simulink model "combined_mdl_wpanel"  (R2024b)
settings: Solver=FixedStepAuto  StartTime=0.0  StopTime=Inf  FixedStep=0.1  MaxStep=1e-3  RelTol=1e-3
model workspace: external: MATLAB File model\combined_mdl_wpanel_wkspc.m (data not in the file)
values from neighbouring files (symbols this model uses):
  sample_period_ms = 100    [combined_mdl_wpanel_wkspc.m]
undefined symbols (not defined in the file or in its folder): DiscIntNeverNeededParam, Serial_Port, Standard_Devices
libraries: simulink x2, sldrtlib x2
settings Model: Creator=apm3  LastModifiedBy=baley
settings HardwareCC: ProdBitPerLong=64  ProdHWDeviceType=Intel->x86-64 (Linux 64)
settings ModelReferenceCC: EnableRefExpFcnMdlSchedulingChecks=on
settings RTWCC: Description=Simulink Desktop Real-Time  SystemTargetFile=sldrt.tlc  TemplateMakefile=sldrt.tmf  RTWCompilerOptimization=on  GPUComputeCapability=3.5
settings CodeAppCC: MaxIdLength=95
settings SimulinkDesktopRealTimeCC: TargetLibSuffix=_sldrt.a  TargetPreCompLibLocation=/home/baley/matlab/R2024b/toolbox/sldrt/lib/glnxa64  ParMdlRefBuildCompliant=on

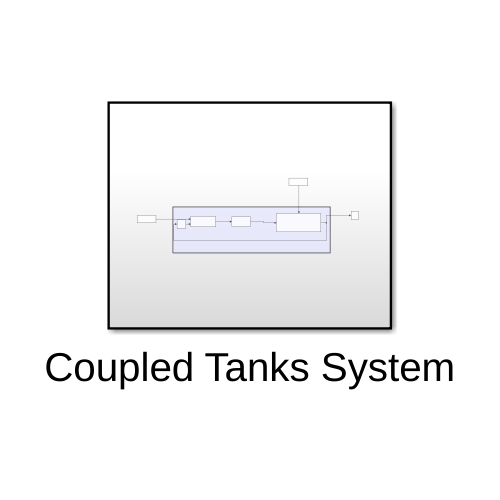
[thumbnail: Simulink's stored preview of the top-level diagram]
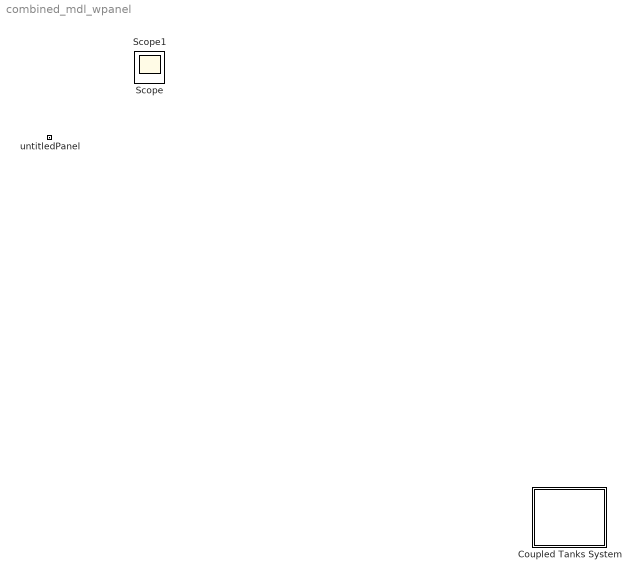
== system combined_mdl_wpanel ==
  Coupled Tanks System : Subsystem
  untitledPanel : Subsystem  Tag=HiddenForWebPanel  IsWebBlockPanel=on
  Scope : Scope
  Scope1 : Scope

== system combined_mdl_wpanel/Coupled Tanks System ==
  note: System
  Controller : Subsystem
  Disturbance : Subsystem
      settings: PortSchema="{\"entries\":[{\"content\":{\"sides\":[{\"content\":{},\"type\":\"ConnectorPlacement.EquallySpacedRectSide\",\"uuid\":\"af3cbaf0-e8cb-4094-98c2-a613e4267cda\"},{\"content\":{\"side\":\"RIGHT\"},\"type\":\"ConnectorPlacement.EquallySpacedRectSide\",\"uuid\":\"ca2a579d-f09d-4edc-8bb1-bcf470cd6e52\"},{\"content\":{\"side\":\"TOP\"},\"type\":\"ConnectorPlacement.EquallySpacedRectSide\",\"uuid\":\"8ccf8dff-0f76-45f4-a120-4302248ce1f5\"},{\"content\":{\"connectorIds\":[\"Out1\"],\"side\":\"BOTTOM\"},\"type\":\"ConnectorPlacement.EquallySpacedRectSide\",\"uuid\":\"e11fb4df-eb62-4915-8053-08a1cec1e132\"}]},\"type\":\"ConnectorPlacement.EquallySpacedConnector\",\"uuid\":\"71d40907-b541-4068-8366-dc0e6cb107c2\"}],\"packageUris\":[\"http://schema.mathworks.com/mf0/Connector/R2020b\"],\"version\":\"1.0\"}"
  Feedback : Subsystem
  Output Scope : Scope
  Plant - Coupled Tanks : Subsystem
      settings: PortSchema="{\"entries\":[{\"content\":{\"sides\":[{\"content\":{\"connectorIds\":[\"In1\"]},\"type\":\"ConnectorPlacement.EquallySpacedRectSide\",\"uuid\":\"4813ac87-9876-4add-8b68-135f8eb15e0b\"},{\"content\":{\"connectorIds\":[\"Out1\"],\"side\":\"RIGHT\"},\"type\":\"ConnectorPlacement.EquallySpacedRectSide\",\"uuid\":\"8da6c8ab-654d-4da4-994c-054b6b84e45c\"},{\"content\":{\"connectorIds\":[\"In2\"],\"side\":\"TOP\"},\"type\":\"ConnectorPlacement.EquallySpacedRectSide\",\"uuid\":\"bc816fc0-ca42-463e-8b06-f8322ae18973\"},{\"content\":{\"side\":\"BOTTOM\"},\"type\":\"ConnectorPlacement.EquallySpacedRectSide\",\"uuid\":\"34484812-162f-4898-b397-ade1a8525c9d\"}]},\"type\":\"ConnectorPlacement.EquallySpacedConnector\",\"uuid\":\"89f4005a-211d-406b-8623-1dc8ebdf98c9\"}],\"packageUris\":[\"http://schema.mathworks.com/mf0/Connector/R2020b\"],\"version\":\"1.0\"}"
  Reference Signal : Subsystem
  Unit Delay : UnitDelay  SampleTime=-1  HasFrameUpgradeWarning=on
  wires:
  Controller/1(Controller Output) -> Plant - Coupled Tanks/1(In2)
  Plant - Coupled Tanks/1(Output Variable) -> Output Scope/1, Unit Delay/1  "measured"
  Disturbance/1(Disturbance Signal) -> Plant - Coupled Tanks/2(Disturbance)
  Reference Signal/1(Reference Signal) -> Feedback/1(Signal)
  Feedback/1(Output) -> Controller/1(Input)
  Unit Delay/1 -> Feedback/2(Output Variable)

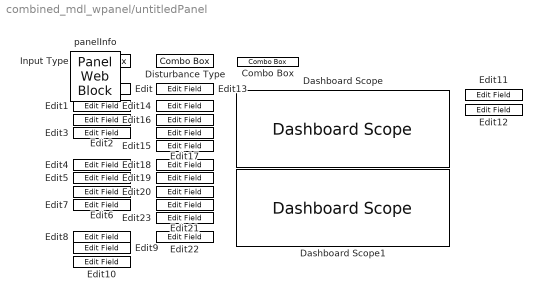
== system combined_mdl_wpanel/untitledPanel ==
  Combo Box : ComboBox  Tag=HiddenForWebPanel  PanelInfo="{\"height\":19,\"left\":400,\"panelId\":\"panelId-cfd753c6-38f0-4228-886e-ef133e3498b9\",\"top\":46,\"type\":\"panelChild\",\"version\":\"2019b\",\"width\":134,\"zIndex\":1500004}"  LabelPosition=Hide  SelectedLabel=Actual Plant
      settings: Values={{'Simulated Plant', 'Actual Plant'}, [0 1]}
  Dashboard Scope : DashboardScope  Tag=HiddenForWebPanel  PanelInfo="{\"height\":168,\"left\":397,\"panelId\":\"panelId-cfd753c6-38f0-4228-886e-ef133e3498b9\",\"top\":119,\"type\":\"panelChild\",\"version\":\"2019b\",\"width\":467,\"zIndex\":1500010}"
  Dashboard Scope1 : DashboardScope  Tag=HiddenForWebPanel  PanelInfo="{\"height\":168,\"left\":397,\"panelId\":\"panelId-cfd753c6-38f0-4228-886e-ef133e3498b9\",\"top\":292,\"type\":\"panelChild\",\"version\":\"2019b\",\"width\":467,\"zIndex\":1500058}"
  Disturbance Type : ComboBox  Tag=HiddenForWebPanel  PanelInfo="{\"height\":29,\"left\":222,\"panelId\":\"panelId-cfd753c6-38f0-4228-886e-ef133e3498b9\",\"top\":40,\"type\":\"panelChild\",\"version\":\"2019b\",\"width\":125,\"zIndex\":1500006}"  LabelPosition=Hide  SelectedLabel=None
      settings: Values={{'None', 'Constant', 'Sine', 'Square', 'Chirp', 'Arbitrary'}, [1 2 3 4 5 6]}
  Edit : EditField  Tag=HiddenForWebPanel  PanelInfo="{\"height\":24,\"left\":40,\"panelId\":\"panelId-cfd753c6-38f0-4228-886e-ef133e3498b9\",\"top\":103,\"type\":\"panelChild\",\"version\":\"2019b\",\"width\":125,\"zIndex\":1500018}"  ShowInitialText=on  Alignment=Left
  Edit1 : EditField  Tag=HiddenForWebPanel  PanelInfo="{\"height\":24,\"left\":40,\"panelId\":\"panelId-cfd753c6-38f0-4228-886e-ef133e3498b9\",\"top\":141,\"type\":\"panelChild\",\"version\":\"2019b\",\"width\":125,\"zIndex\":1500008}"  ShowInitialText=on  Alignment=Left
  Edit10 : EditField  Tag=HiddenForWebPanel  PanelInfo="{\"height\":24,\"left\":40,\"panelId\":\"panelId-cfd753c6-38f0-4228-886e-ef133e3498b9\",\"top\":482,\"type\":\"panelChild\",\"version\":\"2019b\",\"width\":125,\"zIndex\":1500040}"  ShowInitialText=on  Alignment=Left
  Edit11 : EditField  Tag=HiddenForWebPanel  PanelInfo="{\"height\":24,\"left\":900,\"panelId\":\"panelId-cfd753c6-38f0-4228-886e-ef133e3498b9\",\"top\":116,\"type\":\"panelChild\",\"version\":\"2019b\",\"width\":125,\"zIndex\":1500046}"  ShowInitialText=on  Alignment=Left
  Edit12 : EditField  Tag=HiddenForWebPanel  PanelInfo="{\"height\":24,\"left\":900,\"panelId\":\"panelId-cfd753c6-38f0-4228-886e-ef133e3498b9\",\"top\":149,\"type\":\"panelChild\",\"version\":\"2019b\",\"width\":125,\"zIndex\":1500048}"  ShowInitialText=on  Alignment=Left
  Edit13 : EditField  Tag=HiddenForWebPanel  PanelInfo="{\"height\":24,\"left\":222,\"panelId\":\"panelId-cfd753c6-38f0-4228-886e-ef133e3498b9\",\"top\":103,\"type\":\"panelChild\",\"version\":\"2019b\",\"width\":125,\"zIndex\":1500024}"  ShowInitialText=on  Alignment=Left
  Edit14 : EditField  Tag=HiddenForWebPanel  PanelInfo="{\"height\":24,\"left\":222,\"panelId\":\"panelId-cfd753c6-38f0-4228-886e-ef133e3498b9\",\"top\":141,\"type\":\"panelChild\",\"version\":\"2019b\",\"width\":125,\"zIndex\":1500042}"  ShowInitialText=on  Alignment=Left
  Edit15 : EditField  Tag=HiddenForWebPanel  PanelInfo="{\"height\":24,\"left\":222,\"panelId\":\"panelId-cfd753c6-38f0-4228-886e-ef133e3498b9\",\"top\":228,\"type\":\"panelChild\",\"version\":\"2019b\",\"width\":125,\"zIndex\":1500028}"  ShowInitialText=on  Alignment=Left
  Edit16 : EditField  Tag=HiddenForWebPanel  PanelInfo="{\"height\":24,\"left\":222,\"panelId\":\"panelId-cfd753c6-38f0-4228-886e-ef133e3498b9\",\"top\":171,\"type\":\"panelChild\",\"version\":\"2019b\",\"width\":125,\"zIndex\":1500020}"  ShowInitialText=on  Alignment=Left
  Edit17 : EditField  Tag=HiddenForWebPanel  PanelInfo="{\"height\":24,\"left\":222,\"panelId\":\"panelId-cfd753c6-38f0-4228-886e-ef133e3498b9\",\"top\":200,\"type\":\"panelChild\",\"version\":\"2019b\",\"width\":125,\"zIndex\":1500002}"  ShowInitialText=on  Alignment=Left
  Edit18 : EditField  Tag=HiddenForWebPanel  PanelInfo="{\"height\":24,\"left\":222,\"panelId\":\"panelId-cfd753c6-38f0-4228-886e-ef133e3498b9\",\"top\":269,\"type\":\"panelChild\",\"version\":\"2019b\",\"width\":125,\"zIndex\":1500030}"  ShowInitialText=on  Alignment=Left
  Edit19 : EditField  Tag=HiddenForWebPanel  PanelInfo="{\"height\":24,\"left\":222,\"panelId\":\"panelId-cfd753c6-38f0-4228-886e-ef133e3498b9\",\"top\":298,\"type\":\"panelChild\",\"version\":\"2019b\",\"width\":125,\"zIndex\":1500032}"  ShowInitialText=on  Alignment=Left
  Edit2 : EditField  Tag=HiddenForWebPanel  PanelInfo="{\"height\":24,\"left\":40,\"panelId\":\"panelId-cfd753c6-38f0-4228-886e-ef133e3498b9\",\"top\":171,\"type\":\"panelChild\",\"version\":\"2019b\",\"width\":125,\"zIndex\":1500026}"  ShowInitialText=on  Alignment=Left
  Edit20 : EditField  Tag=HiddenForWebPanel  PanelInfo="{\"height\":24,\"left\":222,\"panelId\":\"panelId-cfd753c6-38f0-4228-886e-ef133e3498b9\",\"top\":328,\"type\":\"panelChild\",\"version\":\"2019b\",\"width\":125,\"zIndex\":1500044}"  ShowInitialText=on  Alignment=Left
  Edit21 : EditField  Tag=HiddenForWebPanel  PanelInfo="{\"height\":24,\"left\":222,\"panelId\":\"panelId-cfd753c6-38f0-4228-886e-ef133e3498b9\",\"top\":357,\"type\":\"panelChild\",\"version\":\"2019b\",\"width\":125,\"zIndex\":1500012}"  ShowInitialText=on  Alignment=Left
  Edit22 : EditField  Tag=HiddenForWebPanel  PanelInfo="{\"height\":24,\"left\":222,\"panelId\":\"panelId-cfd753c6-38f0-4228-886e-ef133e3498b9\",\"top\":428,\"type\":\"panelChild\",\"version\":\"2019b\",\"width\":125,\"zIndex\":1500014}"  ShowInitialText=on  Alignment=Left
  Edit23 : EditField  Tag=HiddenForWebPanel  PanelInfo="{\"height\":24,\"left\":222,\"panelId\":\"panelId-cfd753c6-38f0-4228-886e-ef133e3498b9\",\"top\":385,\"type\":\"panelChild\",\"version\":\"2019b\",\"width\":125,\"zIndex\":1500034}"  ShowInitialText=on  Alignment=Left
  Edit3 : EditField  Tag=HiddenForWebPanel  PanelInfo="{\"height\":24,\"left\":40,\"panelId\":\"panelId-cfd753c6-38f0-4228-886e-ef133e3498b9\",\"top\":200,\"type\":\"panelChild\",\"version\":\"2019b\",\"width\":125,\"zIndex\":1500016}"  ShowInitialText=on  Alignment=Left
  Edit4 : EditField  Tag=HiddenForWebPanel  PanelInfo="{\"height\":24,\"left\":40,\"panelId\":\"panelId-cfd753c6-38f0-4228-886e-ef133e3498b9\",\"top\":269,\"type\":\"panelChild\",\"version\":\"2019b\",\"width\":125,\"zIndex\":1500036}"  ShowInitialText=on  Alignment=Left
  Edit5 : EditField  Tag=HiddenForWebPanel  PanelInfo="{\"height\":24,\"left\":40,\"panelId\":\"panelId-cfd753c6-38f0-4228-886e-ef133e3498b9\",\"top\":298,\"type\":\"panelChild\",\"version\":\"2019b\",\"width\":125,\"zIndex\":1500022}"  ShowInitialText=on  Alignment=Left
  Edit6 : EditField  Tag=HiddenForWebPanel  PanelInfo="{\"height\":24,\"left\":40,\"panelId\":\"panelId-cfd753c6-38f0-4228-886e-ef133e3498b9\",\"top\":328,\"type\":\"panelChild\",\"version\":\"2019b\",\"width\":125,\"zIndex\":1500038}"  ShowInitialText=on  Alignment=Left
  Edit7 : EditField  Tag=HiddenForWebPanel  PanelInfo="{\"height\":24,\"left\":40,\"panelId\":\"panelId-cfd753c6-38f0-4228-886e-ef133e3498b9\",\"top\":357,\"type\":\"panelChild\",\"version\":\"2019b\",\"width\":125,\"zIndex\":1500050}"  ShowInitialText=on  Alignment=Left
  Edit8 : EditField  Tag=HiddenForWebPanel  PanelInfo="{\"height\":24,\"left\":40,\"panelId\":\"panelId-cfd753c6-38f0-4228-886e-ef133e3498b9\",\"top\":428,\"type\":\"panelChild\",\"version\":\"2019b\",\"width\":125,\"zIndex\":1500054}"  ShowInitialText=on  Alignment=Left
  Edit9 : EditField  Tag=HiddenForWebPanel  PanelInfo="{\"height\":24,\"left\":40,\"panelId\":\"panelId-cfd753c6-38f0-4228-886e-ef133e3498b9\",\"top\":452,\"type\":\"panelChild\",\"version\":\"2019b\",\"width\":125,\"zIndex\":1500056}"  ShowInitialText=on  Alignment=Left
  Input Type : ComboBox  Tag=HiddenForWebPanel  PanelInfo="{\"height\":29,\"left\":40,\"panelId\":\"panelId-cfd753c6-38f0-4228-886e-ef133e3498b9\",\"top\":40,\"type\":\"panelChild\",\"version\":\"2019b\",\"width\":125,\"zIndex\":1500052}"  LabelPosition=Hide  SelectedLabel=None
      settings: Values={{'None', 'Constant', 'Sine', 'Square', 'Chirp', 'Arbitrary'}, [1 2 3 4 5 6]}
  panelInfo : PanelWebBlock  Tag=HiddenForWebPanel  PanelInfo="{\"compacted\":false,\"height\":557,\"isActiveTab\":true,\"left\":13,\"name\":\"Panel\",\"panelId\":\"panelId-cfd753c6-38f0-4228-886e-ef133e3498b9\",\"popoutData\":{\"height\":1161,\"left\":-1,\"maximized\":false,\"top\":-8,\"width\":1922},\"popoutMode\":\"windowHidden\",\"tabIndex\":0,\"tabbedSetId\":\"tabbedSet6961756998\",\"top\":50,\"type\":\"panel\",\"version\":\"2019b\",\"visible\":true,\"width\":1077,\"zIndex\":1500002}"  PanelSnapshot=<binary blob, 93600 chars, not shown>

== system combined_mdl_wpanel/Coupled Tanks System/Controller ==
  Input : Inport
  To Workspace : ToWorkspace  VariableName=control_output  SaveFormat=Timeseries  SampleTime=-1
  Controller Output : Outport
  wires:
  Input/1 -> To Workspace/1, Controller Output/1

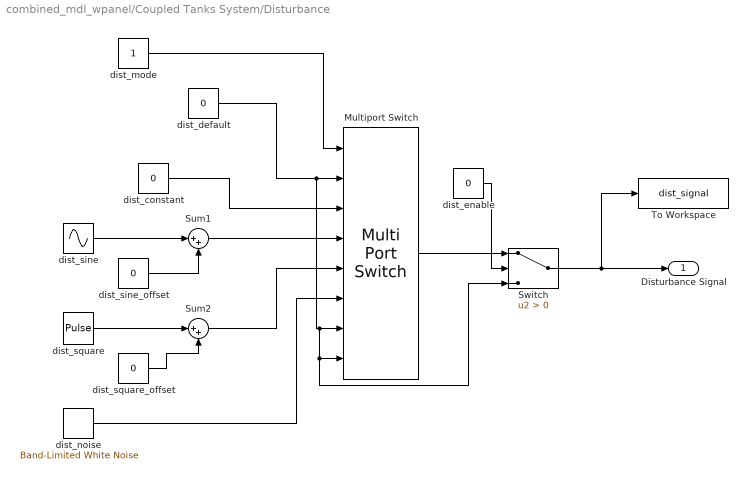
== system combined_mdl_wpanel/Coupled Tanks System/Disturbance ==
  Multiport Switch : MultiPortSwitch  Inputs=6  DataPortForDefault=Additional data port  SaturateOnIntegerOverflow=off  InputSameDT=off
  Sum1 : Sum  Inputs=|++
  Sum2 : Sum  Inputs=|++
  Switch : Switch  Criteria=u2 > Threshold  SaturateOnIntegerOverflow=off  InputSameDT=off
  To Workspace : ToWorkspace  VariableName=dist_signal  SaveFormat=Timeseries  SampleTime=-1
  dist_constant : Constant  Value=0
  dist_default : Constant  Value=0
  dist_enable : Constant  Value=0
  dist_mode : Constant
  dist_noise : simulink/Sources/Band-Limited White Noise  Cov=0  Ts=0.1  seed=[23341]
  dist_sine : Sin  Amplitude=0  Frequency=0  SampleTime=0
  dist_sine_offset : Constant  Value=0
  dist_square : DiscretePulseGenerator  PulseType=Time based  Amplitude=0  Period=1  PulseWidth=50
  dist_square_offset : Constant  Value=0
  Disturbance Signal : Outport
  wires:
  dist_sine/1 -> Sum1/1
  dist_sine_offset/1 -> Sum1/2
  dist_square_offset/1 -> Sum2/2
  dist_square/1 -> Sum2/1
  dist_mode/1 -> Multiport Switch/1
  dist_constant/1 -> Multiport Switch/3
  Sum1/1 -> Multiport Switch/4
  Sum2/1 -> Multiport Switch/5
  dist_noise/1 -> Multiport Switch/6
  Switch/1 -> To Workspace/1, Disturbance Signal/1
  dist_default/1 -> Multiport Switch/8, Switch/3, Multiport Switch/7, Multiport Switch/2
  Multiport Switch/1 -> Switch/1
  dist_enable/1 -> Switch/2

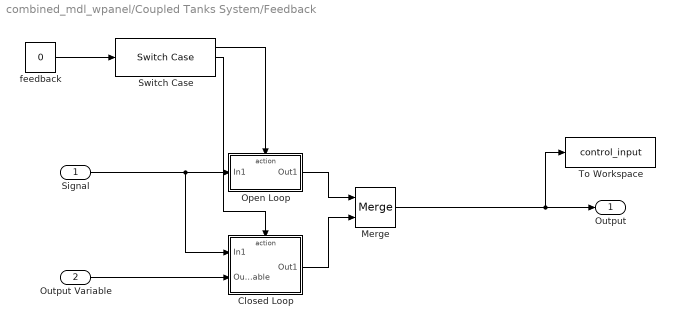
== system combined_mdl_wpanel/Coupled Tanks System/Feedback ==
  Signal : Inport
  Output Variable : Inport  Port=2
  Closed Loop : Subsystem  TreatAsAtomicUnit=on
  Merge : Merge
  Open Loop : Subsystem  TreatAsAtomicUnit=on
  Switch Case : SwitchCase  CaseConditions={0,1}
  To Workspace : ToWorkspace  VariableName=control_input  SaveFormat=Timeseries  SampleTime=-1
  feedback : Constant  Value=0
  Output : Outport
  wires:
  Output Variable/1 -> Closed Loop/2(Output Variable)
  Switch Case/1 -> Open Loop/Action
  Merge/1 -> To Workspace/1, Output/1
  Closed Loop/1(Out1) -> Merge/2
  feedback/1 -> Switch Case/1
  Open Loop/1(Out1) -> Merge/1
  Signal/1 -> Closed Loop/1(In1), Open Loop/1(In1)
  Switch Case/2 -> Closed Loop/Action

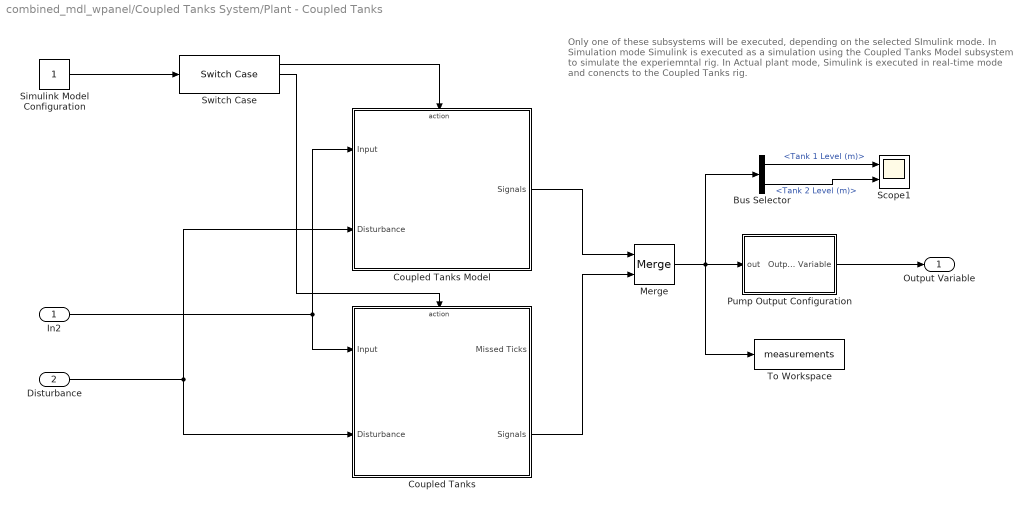
== system combined_mdl_wpanel/Coupled Tanks System/Plant - Coupled Tanks ==
  note: Only one of these subsystems will be executed, depending on the selected SImulink mode.
      |
      | In Simulation mode Simulink is executed as a simulation using the Coupled Tanks Model subsystem to simulate the experiemntal rig.
      |
      | In Actual plant mode, Simulink is executed in real-time mode and conencts to the Coupled Tanks rig.
  In2 : Inport
  Disturbance : Inport  Port=2
  Bus Selector : BusSelector  OutputSignals=Tank 1 Level (m),Tank 2 Level (m)
  Coupled Tanks : Subsystem  TreatAsAtomicUnit=on
  Coupled Tanks Model : Subsystem  TreatAsAtomicUnit=on
  Merge : Merge
  Pump Output Configuration : Subsystem
  Scope1 : Scope  NumInputPorts=2
  Simulink Model Configuration : Constant  OutMin=0  OutMax=1  OutDataTypeStr=int8
  Switch Case : SwitchCase  CaseConditions={0, 1}
  To Workspace : ToWorkspace  VariableName=measurements  SaveFormat=Timeseries  SampleTime=-1
  Output Variable : Outport
  wires:
  Switch Case/2 -> Coupled Tanks/Action
  Switch Case/1 -> Coupled Tanks Model/Action
  In2/1 -> Coupled Tanks/1(Input), Coupled Tanks Model/1(Input)
  Simulink Model Configuration/1 -> Switch Case/1
  Coupled Tanks Model/1(Signals) -> Merge/1
  Coupled Tanks/2(Signals) -> Merge/2
  Merge/1 -> To Workspace/1, Bus Selector/1, Pump Output Configuration/1(out)
  Disturbance/1 -> Coupled Tanks Model/2(Disturbance), Coupled Tanks/2(Disturbance)
  Pump Output Configuration/1(Output Variable) -> Output Variable/1
  Bus Selector/1 -> Scope1/1  "<Tank 1 Level (m)>"
  Bus Selector/2 -> Scope1/2  "<Tank 2 Level (m)>"

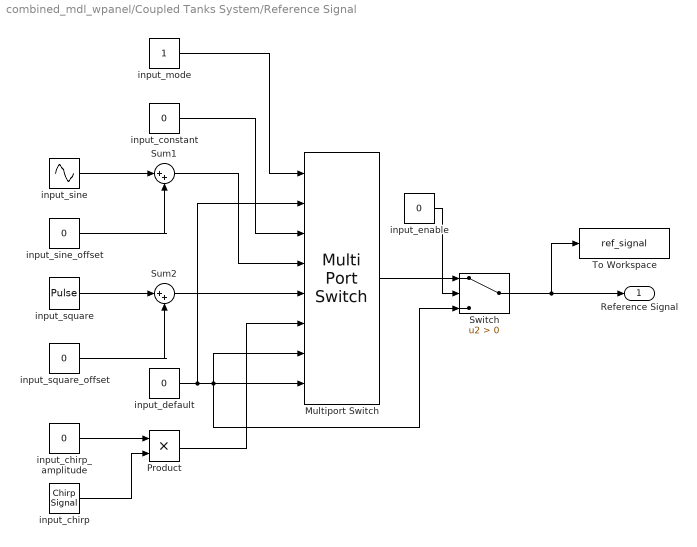
== system combined_mdl_wpanel/Coupled Tanks System/Reference Signal ==
  Multiport Switch : MultiPortSwitch  Inputs=6  DataPortForDefault=Additional data port  SaturateOnIntegerOverflow=off  InputSameDT=off
  Product : Product
  Sum1 : Sum  Inputs=|++
  Sum2 : Sum  Inputs=|++
  Switch : Switch  Criteria=u2 > Threshold  SaturateOnIntegerOverflow=off  InputSameDT=off
  To Workspace : ToWorkspace  VariableName=ref_signal  SaveFormat=Timeseries  SampleTime=-1
  input_chirp : simulink/Sources/Chirp Signal  f1=0  T=0  f2=0
  input_chirp_amplitude : Constant  Value=0
  input_constant : Constant  Value=0
  input_default : Constant  Value=0
  input_enable : Constant  Value=0
  input_mode : Constant
  input_sine : Sin  Amplitude=0  Frequency=0  SampleTime=0
  input_sine_offset : Constant  Value=0
  input_square : DiscretePulseGenerator  PulseType=Time based  Amplitude=0  Period=1  PulseWidth=50
  input_square_offset : Constant  Value=0
  Reference Signal : Outport
  wires:
  input_constant/1 -> Multiport Switch/3
  input_mode/1 -> Multiport Switch/1
  input_square_offset/1 -> Sum2/2
  input_chirp/1 -> Product/2
  input_chirp_amplitude/1 -> Product/1
  Sum2/1 -> Multiport Switch/5
  input_square/1 -> Sum2/1
  input_sine_offset/1 -> Sum1/2
  Sum1/1 -> Multiport Switch/4
  input_sine/1 -> Sum1/1
  input_default/1 -> Switch/3, Multiport Switch/8, Multiport Switch/7, Multiport Switch/2
  Product/1 -> Multiport Switch/6
  Switch/1 -> To Workspace/1, Reference Signal/1
  Multiport Switch/1 -> Switch/1
  input_enable/1 -> Switch/2

== system combined_mdl_wpanel/Coupled Tanks System/Feedback/Closed Loop ==
  In1 : Inport
  Output Variable : Inport  Port=2
  Action Port : ActionPort  ActionPortLabel=case [ 1 ]:
  Sum : Sum  Inputs=|+-
  Out1 : Outport
  wires:
  Output Variable/1 -> Sum/2
  In1/1 -> Sum/1
  Sum/1 -> Out1/1

== system combined_mdl_wpanel/Coupled Tanks System/Feedback/Open Loop ==
  In1 : Inport
  Action Port : ActionPort  ActionPortLabel=case [ 0 ]:
  Out1 : Outport
  wires:
  In1/1 -> Out1/1

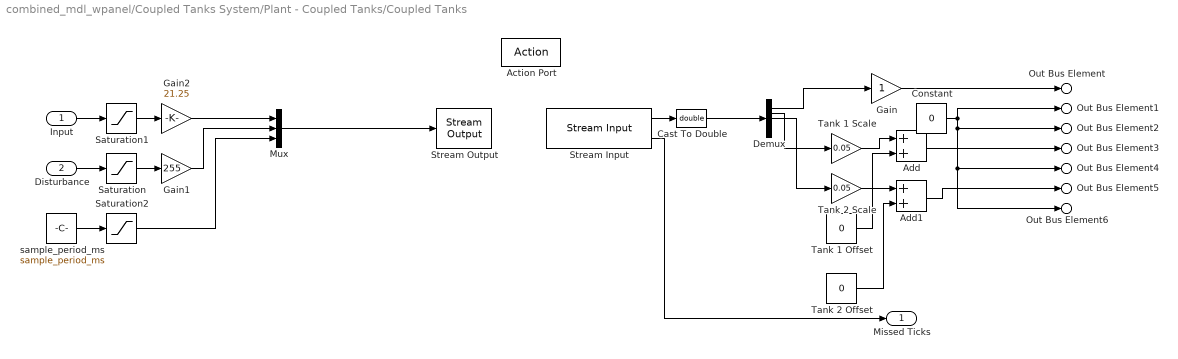
== system combined_mdl_wpanel/Coupled Tanks System/Plant - Coupled Tanks/Coupled Tanks ==
  Input : Inport
  Disturbance : Inport  Port=2
  Action Port : ActionPort  ActionPortLabel=case [ 1 ]:
  Add : Sum
  Add1 : Sum
  Cast To Double : DataTypeConversion  OutDataTypeStr=double  SaturateOnIntegerOverflow=off  RndMeth=Floor
  Constant : Constant  Value=0
  Demux : Demux  Outputs=5
  Gain : Gain
  Gain1 : Gain  Gain=255
  Gain2 : Gain  Gain=21.25
  Mux : Mux  Inputs=3
  Saturation : Saturate  UpperLimit=1  LowerLimit=0
  Saturation1 : Saturate  UpperLimit=12  LowerLimit=0
  Saturation2 : Saturate  UpperLimit=1000  LowerLimit=0
  Stream Input : sldrtlib/Stream Input  SampleTime=0.1  MaxMissedTicks=50  ShowMissedTicks=on  YieldWhenWaiting=on  DrvName=Standard_Devices/Serial_Port  DrvAddress=12  DrvOptions=[9600 8 0 0 0 0 0 0]  DataTypes='5*int16'  FormatString='%d,%d,%d,%d,%d'  Terminator={'\n'}  ShowReady=off  ShowError=off
      settings: AttributesFormatString=Serial Port [10]
  Stream Output : sldrtlib/Stream Output  SampleTime=0.1  MaxMissedTicks=10  ShowMissedTicks=off  YieldWhenWaiting=off  DrvName=Standard_Devices/Serial_Port  DrvAddress=12  DrvOptions=[9600 8 0 0 0 0 0 0]  PortSizes=3  FormatString='%d,%d,%d\n'  ShowReady=off  ShowError=off  InitialValue=[]  FinalValue=[]
      settings: AttributesFormatString=Serial Port [10]
  Tank 1 Offset : Constant  Value=0
  Tank 1 Scale : Gain  Gain=0.05
  Tank 2 Offset : Constant  Value=0
  Tank 2 Scale : Gain  Gain=0.05
  sample_period_ms : Constant  Value=sample_period_ms  VectorParams1D=off
  Missed Ticks : Outport
  Out Bus Element : Outport  Port=2  PortName=Signals  Element=Pump Current (A)
  Out Bus Element1 : Outport  Port=2  PortName=Signals  Element=Out 1 Flow (L/min)
  Out Bus Element2 : Outport  Port=2  PortName=Signals  Element=Out 2 Flow (L/min)
  Out Bus Element3 : Outport  Port=2  PortName=Signals  Element=Tank 1 Level (m)
  Out Bus Element4 : Outport  Port=2  PortName=Signals  Element=Tank 1 Outlet Flow (L/min)
  Out Bus Element5 : Outport  Port=2  PortName=Signals  Element=Tank 2 Level (m)
  Out Bus Element6 : Outport  Port=2  PortName=Signals  Element=Tank 2 Outlet Flow (L/min)
  wires:
  Stream Input/2 -> Missed Ticks/1
  Stream Input/1 -> Cast To Double/1
  Cast To Double/1 -> Demux/1
  Demux/1 -> Gain/1
  Gain/1 -> Out Bus Element/1
  Demux/2 -> Tank 1 Scale/1
  Demux/3 -> Tank 2 Scale/1
  Constant/1 -> Out Bus Element1/1, Out Bus Element6/1, Out Bus Element4/1, Out Bus Element2/1
  Input/1 -> Saturation1/1
  sample_period_ms/1 -> Saturation2/1
  Mux/1 -> Stream Output/1
  Disturbance/1 -> Saturation/1
  Saturation/1 -> Gain1/1
  Gain1/1 -> Mux/2
  Saturation1/1 -> Gain2/1
  Gain2/1 -> Mux/1
  Saturation2/1 -> Mux/3
  Tank 1 Scale/1 -> Add/1
  Tank 1 Offset/1 -> Add/2
  Add/1 -> Out Bus Element3/1
  Add1/1 -> Out Bus Element5/1
  Tank 2 Scale/1 -> Add1/1
  Tank 2 Offset/1 -> Add1/2

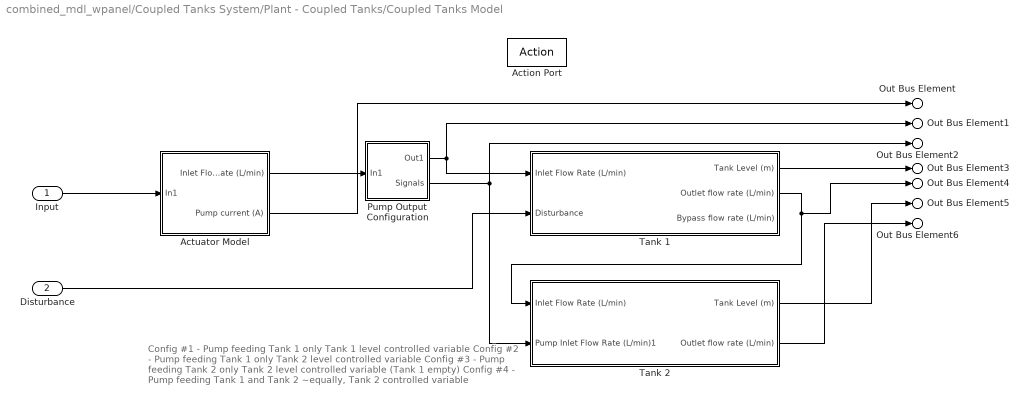
== system combined_mdl_wpanel/Coupled Tanks System/Plant - Coupled Tanks/Coupled Tanks Model ==
  note: Config #1
      | - Pump feeding Tank 1 only Tank 1 level controlled variable
      | Config #2
      | - Pump feeding Tank 1 only Tank 2 level controlled variable
      | Config #3
      | - Pump feeding Tank 2 only Tank 2 level controlled variable (Tank 1 empty)
      | Config #4
      | - Pump feeding Tank 1 and Tank 2 ~equally, Tank 2 controlled variable
  Input : Inport
  Disturbance : Inport  Port=2
  Action Port : ActionPort  ActionPortLabel=case [ 0 ]:
  Actuator Model : Subsystem
  Pump Output Configuration : Subsystem
  Tank 1 : Subsystem
  Tank 2 : Subsystem
  Out Bus Element : Outport  PortName=Signals  Element=Pump Current (A)
  Out Bus Element1 : Outport  PortName=Signals  Element=Out 1 Flow (L/min)
  Out Bus Element2 : Outport  PortName=Signals  Element=Out 2 Flow (L/min)
  Out Bus Element3 : Outport  PortName=Signals  Element=Tank 1 Level (m)
  Out Bus Element4 : Outport  PortName=Signals  Element=Tank 1 Outlet Flow (L/min)
  Out Bus Element5 : Outport  PortName=Signals  Element=Tank 2 Level (m)
  Out Bus Element6 : Outport  PortName=Signals  Element=Tank 2 Outlet Flow (L/min)
  wires:
  Input/1 -> Actuator Model/1(In1)
  Actuator Model/1(Inlet Flow Rate (L/min)) -> Pump Output Configuration/1(In1)
  Tank 1/2(Outlet flow rate (L/min)) -> Tank 2/1(Inlet Flow Rate (L/min)), Out Bus Element4/1
  Tank 1/1(Tank Level (m)) -> Out Bus Element3/1
  Tank 2/1(Tank Level (m)) -> Out Bus Element5/1
  Tank 2/2(Outlet flow rate (L/min)) -> Out Bus Element6/1
  Actuator Model/2(Pump current (A)) -> Out Bus Element/1
  Disturbance/1 -> Tank 1/2(Disturbance)
  Pump Output Configuration/1(Out1) -> Out Bus Element1/1, Tank 1/1(Inlet Flow Rate (L/min))
  Pump Output Configuration/2(Signals) -> Out Bus Element2/1, Tank 2/2(Pump Inlet Flow Rate (L/min)1)

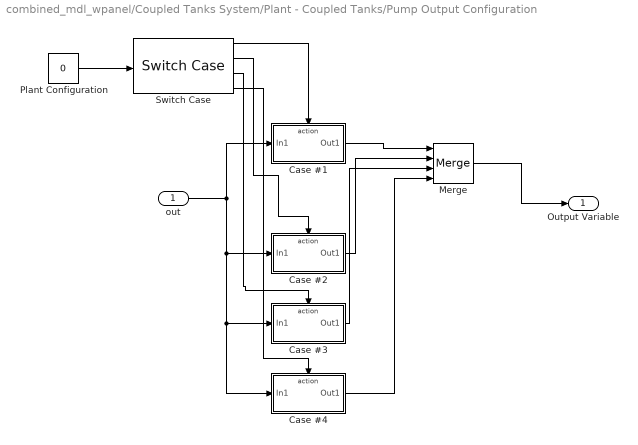
== system combined_mdl_wpanel/Coupled Tanks System/Plant - Coupled Tanks/Pump Output Configuration ==
  out : Inport
  Case #1 : Subsystem  TreatAsAtomicUnit=on
  Case #2 : Subsystem  TreatAsAtomicUnit=on
  Case #3 : Subsystem  TreatAsAtomicUnit=on
  Case #4 : Subsystem  TreatAsAtomicUnit=on
  Merge : Merge  Inputs=4
  Plant Configuration : Constant  Value=0  OutMin=0  OutMax=1  OutDataTypeStr=int8
  Switch Case : SwitchCase  CaseConditions={0, 1, 2, 3}  ShowDefaultCase=off
  Output Variable : Outport
  wires:
  Plant Configuration/1 -> Switch Case/1
  Switch Case/1 -> Case #1/Action
  Switch Case/2 -> Case #2/Action
  Switch Case/3 -> Case #3/Action
  Switch Case/4 -> Case #4/Action
  out/1 -> Case #1/1(In1), Case #2/1(In1), Case #4/1(In1), Case #3/1(In1)
  Case #1/1(Out1) -> Merge/1
  Case #2/1(Out1) -> Merge/2
  Case #3/1(Out1) -> Merge/3
  Merge/1 -> Output Variable/1
  Case #4/1(Out1) -> Merge/4

== system combined_mdl_wpanel/Coupled Tanks System/Plant - Coupled Tanks/Coupled Tanks Model/Actuator Model ==
  note: We assume Volumetric flow at outlet of pump is proportional to the pump voltage
  In1 : Inport
  Kp : Gain  Gain=1/12
  Kp1 : Gain
  Inlet Flow Rate (L/min) : Outport
  Pump current (A) : Outport  Port=2
  wires:
  In1/1 -> Kp/1
  Kp/1 -> Pump current (A)/1, Kp1/1
  Kp1/1 -> Inlet Flow Rate (L/min)/1

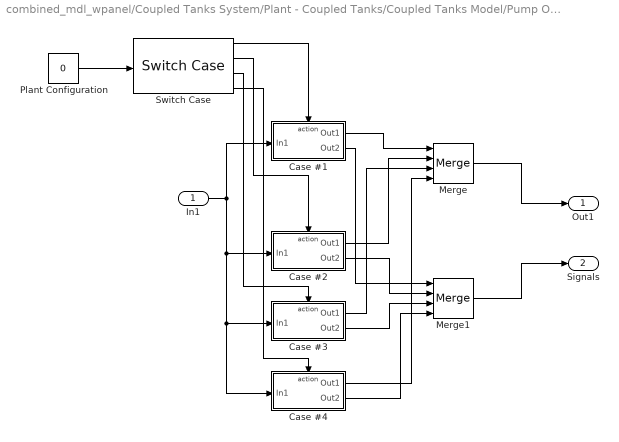
== system combined_mdl_wpanel/Coupled Tanks System/Plant - Coupled Tanks/Coupled Tanks Model/Pump Output Configuration ==
  In1 : Inport
  Case #1 : Subsystem  TreatAsAtomicUnit=on
  Case #2 : Subsystem  TreatAsAtomicUnit=on
  Case #3 : Subsystem  TreatAsAtomicUnit=on
  Case #4 : Subsystem  TreatAsAtomicUnit=on
  Merge : Merge  Inputs=4
  Merge1 : Merge  Inputs=4
  Plant Configuration : Constant  Value=0  OutMin=0  OutMax=1  OutDataTypeStr=int8
  Switch Case : SwitchCase  CaseConditions={0, 1, 2, 3}  ShowDefaultCase=off
  Out1 : Outport
  Signals : Outport  Port=2
  wires:
  Plant Configuration/1 -> Switch Case/1
  Switch Case/1 -> Case #1/Action
  Switch Case/2 -> Case #2/Action
  Switch Case/3 -> Case #3/Action
  Switch Case/4 -> Case #4/Action
  In1/1 -> Case #1/1(In1), Case #4/1(In1), Case #3/1(In1), Case #2/1(In1)
  Case #1/1(Out1) -> Merge/1
  Case #2/1(Out1) -> Merge/2
  Case #3/1(Out1) -> Merge/3
  Case #4/1(Out1) -> Merge/4
  Case #1/2(Out2) -> Merge1/1
  Case #2/2(Out2) -> Merge1/2
  Case #3/2(Out2) -> Merge1/3
  Case #4/2(Out2) -> Merge1/4
  Merge1/1 -> Signals/1
  Merge/1 -> Out1/1

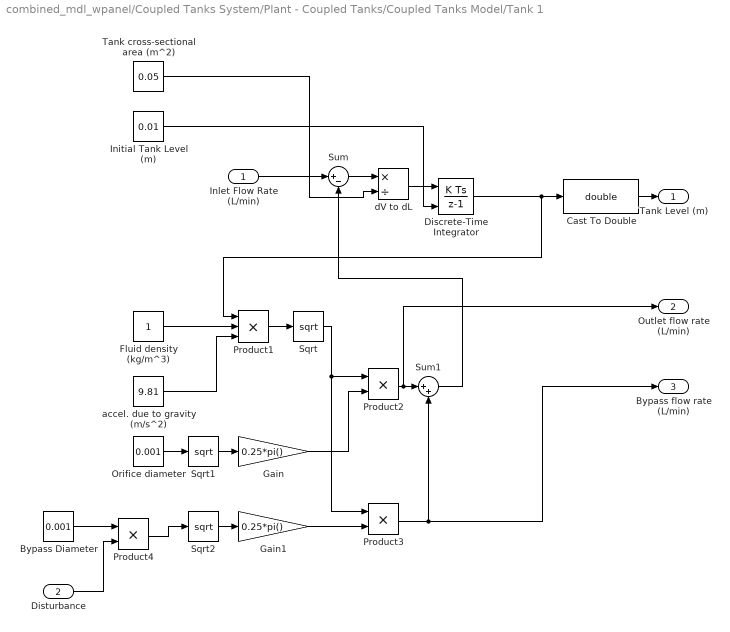
== system combined_mdl_wpanel/Coupled Tanks System/Plant - Coupled Tanks/Coupled Tanks Model/Tank 1 ==
  Inlet Flow Rate (L/min) : Inport
  Disturbance : Inport  Port=2
  Bypass Diameter : Constant  Value=0.001
  Cast To Double : DataTypeConversion  OutDataTypeStr=double  SaturateOnIntegerOverflow=off  RndMeth=Floor
  Discrete-Time Integrator : DiscreteIntegrator  InitialConditionSource=external  SampleTime=-1  LimitOutput=on  UpperSaturationLimit=20  LowerSaturationLimit=0  ICPrevOutput=DiscIntNeverNeededParam  ICPrevScaledInput=DiscIntNeverNeededParam
  Fluid density (kg/m^3) : Constant
  Gain : Gain  Gain=0.25*pi()
  Gain1 : Gain  Gain=0.25*pi()
  Initial Tank Level (m) : Constant  Value=0.01
  Orifice diameter : Constant  Value=0.001
  Product1 : Product  Inputs=3
  Product2 : Product
  Product3 : Product
  Product4 : Product
  Sqrt : Sqrt
  Sqrt1 : Sqrt
  Sqrt2 : Sqrt
  Sum : Sum  Inputs=|+-
  Sum1 : Sum  Inputs=|++
  Tank cross-sectional area (m^2) : Constant  Value=0.05
  accel. due to gravity (m/s^2) : Constant  Value=9.81
  dV to dL : Product  Inputs=*/
  Tank Level (m) : Outport
  Outlet flow rate (L/min) : Outport  Port=2
  Bypass flow rate (L/min) : Outport  Port=3
  wires:
  Inlet Flow Rate (L/min)/1 -> Sum/1
  Discrete-Time Integrator/1 -> Cast To Double/1, Product1/1
  Fluid density (kg/m^3)/1 -> Product1/2
  accel. due to gravity (m/s^2)/1 -> Product1/3
  Product1/1 -> Sqrt/1
  Orifice diameter/1 -> Sqrt1/1
  Sqrt1/1 -> Gain/1
  Sqrt/1 -> Product3/1, Product2/1
  Gain/1 -> Product2/2
  Cast To Double/1 -> Tank Level (m)/1
  Sum/1 -> dV to dL/1
  Tank cross-sectional area (m^2)/1 -> dV to dL/2
  dV to dL/1 -> Discrete-Time Integrator/1
  Initial Tank Level (m)/1 -> Discrete-Time Integrator/2
  Sqrt2/1 -> Gain1/1
  Product2/1 -> Outlet flow rate (L/min)/1, Sum1/1
  Sum1/1 -> Sum/2
  Gain1/1 -> Product3/2
  Product3/1 -> Sum1/2, Bypass flow rate (L/min)/1
  Bypass Diameter/1 -> Product4/1
  Product4/1 -> Sqrt2/1
  Disturbance/1 -> Product4/2

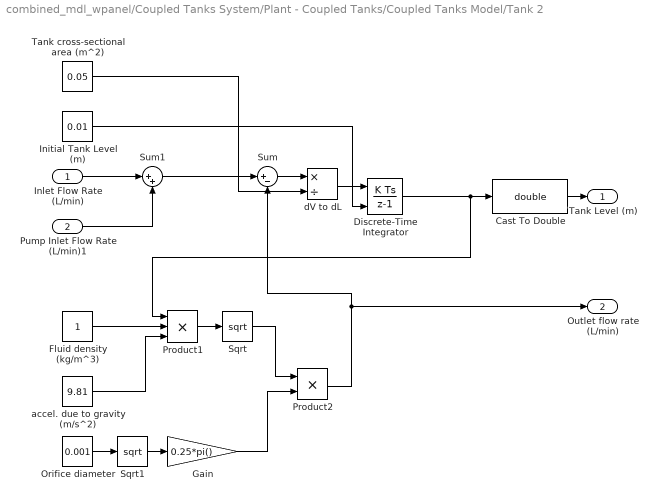
== system combined_mdl_wpanel/Coupled Tanks System/Plant - Coupled Tanks/Coupled Tanks Model/Tank 2 ==
  Inlet Flow Rate (L/min) : Inport
  Pump Inlet Flow Rate (L/min)1 : Inport  Port=2
  Cast To Double : DataTypeConversion  OutDataTypeStr=double  SaturateOnIntegerOverflow=off  RndMeth=Floor
  Discrete-Time Integrator : DiscreteIntegrator  InitialConditionSource=external  SampleTime=-1  LimitOutput=on  UpperSaturationLimit=20  LowerSaturationLimit=0  ICPrevOutput=DiscIntNeverNeededParam  ICPrevScaledInput=DiscIntNeverNeededParam
  Fluid density (kg/m^3) : Constant
  Gain : Gain  Gain=0.25*pi()
  Initial Tank Level (m) : Constant  Value=0.01
  Orifice diameter : Constant  Value=0.001
  Product1 : Product  Inputs=3
  Product2 : Product
  Sqrt : Sqrt
  Sqrt1 : Sqrt
  Sum : Sum  Inputs=|+-
  Sum1 : Sum  Inputs=|++
  Tank cross-sectional area (m^2) : Constant  Value=0.05
  accel. due to gravity (m/s^2) : Constant  Value=9.81
  dV to dL : Product  Inputs=*/
  Tank Level (m) : Outport
  Outlet flow rate (L/min) : Outport  Port=2
  wires:
  Discrete-Time Integrator/1 -> Cast To Double/1, Product1/1
  Fluid density (kg/m^3)/1 -> Product1/2
  accel. due to gravity (m/s^2)/1 -> Product1/3
  Product1/1 -> Sqrt/1
  Orifice diameter/1 -> Sqrt1/1
  Sqrt1/1 -> Gain/1
  Sqrt/1 -> Product2/1
  Gain/1 -> Product2/2
  Product2/1 -> Outlet flow rate (L/min)/1, Sum/2
  Cast To Double/1 -> Tank Level (m)/1
  Sum/1 -> dV to dL/1
  Tank cross-sectional area (m^2)/1 -> dV to dL/2
  dV to dL/1 -> Discrete-Time Integrator/1
  Initial Tank Level (m)/1 -> Discrete-Time Integrator/2
  Inlet Flow Rate (L/min)/1 -> Sum1/1
  Sum1/1 -> Sum/1
  Pump Inlet Flow Rate (L/min)1/1 -> Sum1/2

== system combined_mdl_wpanel/Coupled Tanks System/Plant - Coupled Tanks/Pump Output Configuration/Case #1 ==
  In1 : Inport
  Action Port : ActionPort  ActionPortLabel=case [ 0 ]:
  Bus Selector : BusSelector  OutputSignals=Tank 1 Level (m)
  Out1 : Outport
  wires:
  In1/1 -> Bus Selector/1
  Bus Selector/1 -> Out1/1  "<Tank 1 Level (m)>"

== system combined_mdl_wpanel/Coupled Tanks System/Plant - Coupled Tanks/Pump Output Configuration/Case #2 ==
  In1 : Inport
  Action Port : ActionPort  ActionPortLabel=case [ 1 ]:
  Bus Selector : BusSelector  OutputSignals=Tank 2 Level (m)
  Out1 : Outport
  wires:
  In1/1 -> Bus Selector/1
  Bus Selector/1 -> Out1/1  "<Tank 2 Level (m)>"

== system combined_mdl_wpanel/Coupled Tanks System/Plant - Coupled Tanks/Pump Output Configuration/Case #3 ==
  In1 : Inport
  Action Port : ActionPort  ActionPortLabel=case [ 2 ]:
  Bus Selector : BusSelector  OutputSignals=Tank 2 Level (m)
  Out1 : Outport
  wires:
  In1/1 -> Bus Selector/1
  Bus Selector/1 -> Out1/1  "<Tank 2 Level (m)>"

== system combined_mdl_wpanel/Coupled Tanks System/Plant - Coupled Tanks/Pump Output Configuration/Case #4 ==
  In1 : Inport
  Action Port : ActionPort  ActionPortLabel=case [ 3 ]:
  Bus Selector : BusSelector  OutputSignals=Tank 2 Level (m)
  Out1 : Outport
  wires:
  In1/1 -> Bus Selector/1
  Bus Selector/1 -> Out1/1  "<Tank 2 Level (m)>"

== system combined_mdl_wpanel/Coupled Tanks System/Plant - Coupled Tanks/Coupled Tanks Model/Pump Output Configuration/Case #1 ==
  In1 : Inport
  Action Port : ActionPort  ActionPortLabel=case [ 0 ]:
  Constant : Constant  Value=0
  Out1 : Outport
  Out2 : Outport  Port=2
  wires:
  In1/1 -> Out1/1
  Constant/1 -> Out2/1

== system combined_mdl_wpanel/Coupled Tanks System/Plant - Coupled Tanks/Coupled Tanks Model/Pump Output Configuration/Case #2 ==
  In1 : Inport
  Action Port : ActionPort  ActionPortLabel=case [ 1 ]:
  Constant : Constant  Value=0
  Out1 : Outport
  Out2 : Outport  Port=2
  wires:
  In1/1 -> Out1/1
  Constant/1 -> Out2/1

== system combined_mdl_wpanel/Coupled Tanks System/Plant - Coupled Tanks/Coupled Tanks Model/Pump Output Configuration/Case #3 ==
  In1 : Inport
  Action Port : ActionPort  ActionPortLabel=case [ 2 ]:
  Constant : Constant  Value=0
  Out1 : Outport
  Out2 : Outport  Port=2
  wires:
  Constant/1 -> Out1/1
  In1/1 -> Out2/1

== system combined_mdl_wpanel/Coupled Tanks System/Plant - Coupled Tanks/Coupled Tanks Model/Pump Output Configuration/Case #4 ==
  In1 : Inport
  Action Port : ActionPort  ActionPortLabel=case [ 3 ]:
  Gain : Gain  Gain=0.5
  Out1 : Outport
  Out2 : Outport  Port=2
  wires:
  In1/1 -> Gain/1
  Gain/1 -> Out2/1, Out1/1
